simulink model "nmpc_block_v2015a"  (R2015a)
settings: Solver=ode45  StartTime=0.0  StopTime=10  FixedStep=1  RelTol=1e-3
values from neighbouring files (symbols this model uses):
  K = nmpc_design_st(par)    [nmpc_design_template.m]
settings Model: CovHtmlReporting=off  Creator=carlonovara  LastModifiedBy=carlonovara
settings DataIOCC: LimitDataPoints=off  SaveFormat=Dataset
settings HardwareCC: ProdBitPerPointer=64  ProdLargestAtomicFloat=Float  ProdIntDivRoundTo=Zero  ProdEndianess=LittleEndian  ProdHWDeviceType=Specified
settings ModelReferenceCC: PropagateSignalLabelsOutOfModel=on

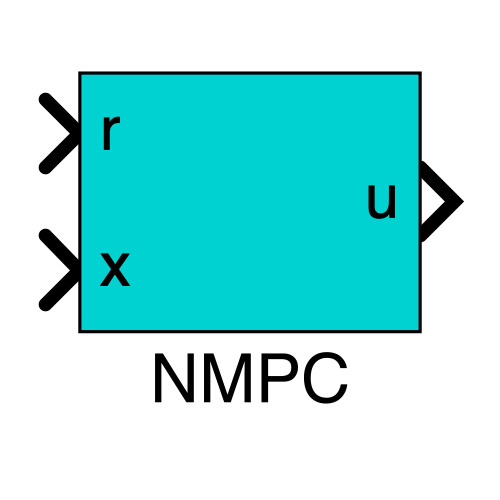
[thumbnail: Simulink's stored preview of the top-level diagram]
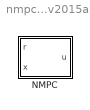
== system nmpc_block_v2015a ==
  NMPC : Subsystem  mask{K=K}
      mask prompts: K "NMPC structure"

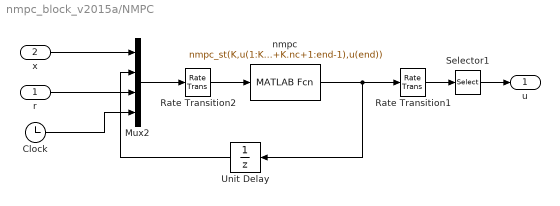
== system nmpc_block_v2015a/NMPC ==
  r : Inport
  x : Inport  Port=2
  Clock : Clock
  Mux2 : Mux
  Rate Transition1 : RateTransition  OutPortSampleTime=K.Ts
  Rate Transition2 : RateTransition  OutPortSampleTime=K.Ts
  Selector1 : Selector  InputPortWidth=K.nc  IndexOptions=Index vector (dialog)  Indices=1:K.nu  OutputSizes=1
  Unit Delay : UnitDelay  InitialCondition=zeros(K.nc,1)  SampleTime=K.Ts  HasFrameUpgradeWarning=on
  nmpc : MATLABFcn  MATLABFcn=nmpc_st(K,u(1:K.nx),u(K.nx+1:K.nx+K.nc),u(K.nx+K.nc+1:end-1),u(end))  OutputDimensions=K.nc
  u : Outport
  wires:
  Selector1/1 -> u/1
  Unit Delay/1 -> Mux2/2
  nmpc/1 -> Unit Delay/1, Rate Transition1/1
  Rate Transition1/1 -> Selector1/1
  Mux2/1 -> Rate Transition2/1
  x/1 -> Mux2/1
  r/1 -> Mux2/3
  Clock/1 -> Mux2/4
  Rate Transition2/1 -> nmpc/1
